simulink model "ROBOT_OK"  (R2021a)
settings: Solver=FixedStepAuto  StartTime=0.0  StopTime=inf  FixedStep=0.001  RelTol=1e-3
model workspace: external: MATLAB File E:\2024\TINH_TOAN_ROBOT_6_DOF\ROBOT_OK_DataFile.m (data not in the file)
values from neighbouring files (symbols this model uses):
  X = Toado(:,1)    [QuydaoK.m]
  Y = Toado(:,2)    [QuydaoK.m]
  Z = Toado(:,3)    [QuydaoK.m]
undefined symbols (not defined in the file or in its folder): smiData
libraries: sm_lib x38, nesl_utility x30, sharedutil x16, sharedtransform x12, dspmtrx3 x12, simulink_extras x8, pid_lib x6, simulink x3
(part 2 of 6)

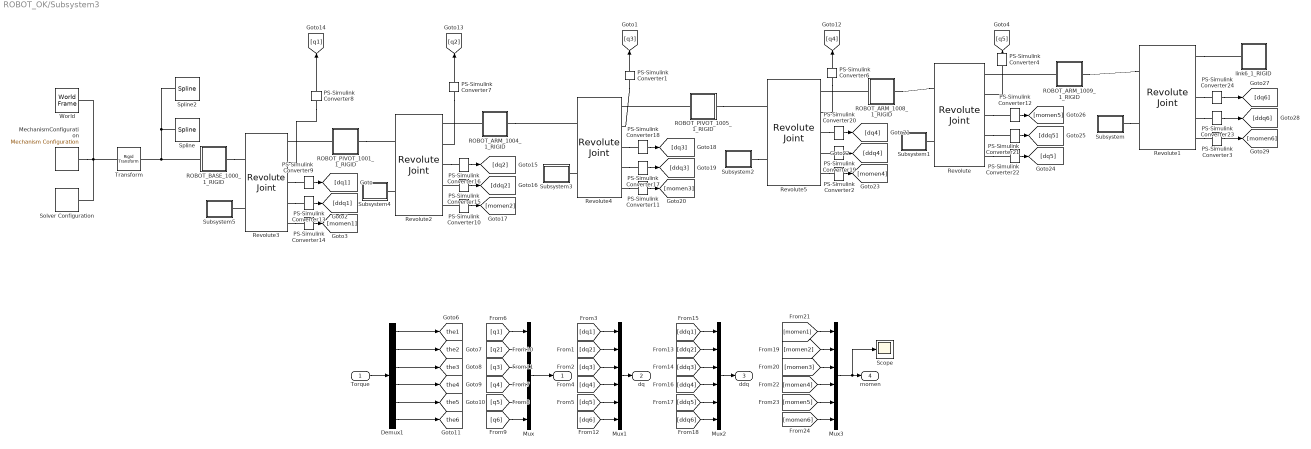
== system ROBOT_OK/Subsystem3 ==
  Torque : Inport
  Demux1 : Demux  Outputs=6
  MechanismConfiguration : sm_lib/Utilities/Mechanism Configuration  UniformGravity=Constant  GravityVector=[0 -9.80665 0]  GravityVectorUnits=m/s^2  GravityUnits=m/s^2  LinearizationDelta=0.001  JointModeTransitionNonlinearIterations=2
  Mux{,1..3} (4 alike) : Mux  Inputs=6
  PS-Simulink Converter{1..4,6..24} (23 alike) : nesl_utility/PS-Simulink Converter  PhysicalDomain=network_engine_domain  SubClassName=ps_output  LeftPortType=input  RightPortType=output  PseudoPeriodic=off  Frequencies=[]  Unit=inherit  AffineConversion=off
      settings: SourceProductBaseCode=PW,SS
  ROBOT_ARM_1004_1_RIGID : Subsystem
  ROBOT_ARM_1008_1_RIGID : Subsystem
  ROBOT_ARM_1009_1_RIGID : Subsystem
  ROBOT_BASE_1000_1_RIGID : Subsystem
  ROBOT_PIVOT_1001_1_RIGID : Subsystem
  ROBOT_PIVOT_1005_1_RIGID : Subsystem
  Revolute : sm_lib/Joints/Revolute Joint  JointMode=Normal  SenseConstraintForce=off  SenseConstraintForceX=off  SenseConstraintForceY=off  SenseConstraintForceZ=off  SenseConstraintTorque=off  SenseConstraintTorqueX=off  SenseConstraintTorqueY=off  SenseConstraintTorqueZ=off  SenseTotalForce=off  SenseTotalForceX=off  SenseTotalForceY=off  SenseTotalForceZ=off  SenseTotalTorque=off  SenseTotalTorqueX=off  SenseTotalTorqueY=off  SenseTotalTorqueZ=off  CompositeWrenchDir=FollowerOnBase  CompositeWrenchFrame=BaseFrame  EquilibriumPosition=0  EquilibriumPositionUnits=deg  SpringStiffness=0  SpringStiffnessUnits=N*m/deg  DampingCoefficient=0  DampingCoefficientUnits=N*m/(deg/s)  TorqueActuationMode=ComputedTorque  MotionActuationMode=InputMotion  SensePosition=on  SenseVelocity=on  SenseAcceleration=on  SenseTorqueForce=on  SenseLowerLimitTorqueForce=off  SenseUpperLimitTorqueForce=off  LowerLimitSpecify=off  LowerLimitBound=-90  LowerLimitBoundUnits=deg  LowerLimitStiffness=1e4  LowerLimitStiffnessUnits=N*m/deg  LowerLimitDamping=10  LowerLimitDampingUnits=N*m/(deg/s)  LowerLimitTransitionRegionWidth=0.1  LowerLimitTransitionRegionWidthUnits=deg  UpperLimitSpecify=off  UpperLimitBound=90  UpperLimitBoundUnits=deg  UpperLimitStiffness=1e4  UpperLimitStiffnessUnits=N*m/deg  UpperLimitDamping=10  UpperLimitDampingUnits=N*m/(deg/s)  UpperLimitTransitionRegionWidth=0.1  UpperLimitTransitionRegionWidthUnits=deg  PositionTargetSpecify=on  PositionTargetPriority=Low  PositionTargetValue=smiData.RevoluteJoint(1).Rz.Pos  PositionTargetValueUnits=deg  VelocityTargetSpecify=off  VelocityTargetPriority=High  VelocityTargetValue=0  VelocityTargetValueUnits=deg/s
  Revolute1 : sm_lib/Joints/Revolute Joint  JointMode=Normal  SenseConstraintForce=off  SenseConstraintForceX=off  SenseConstraintForceY=off  SenseConstraintForceZ=off  SenseConstraintTorque=off  SenseConstraintTorqueX=off  SenseConstraintTorqueY=off  SenseConstraintTorqueZ=off  SenseTotalForce=off  SenseTotalForceX=off  SenseTotalForceY=off  SenseTotalForceZ=off  SenseTotalTorque=off  SenseTotalTorqueX=off  SenseTotalTorqueY=off  SenseTotalTorqueZ=off  CompositeWrenchDir=FollowerOnBase  CompositeWrenchFrame=BaseFrame  EquilibriumPosition=0  EquilibriumPositionUnits=deg  SpringStiffness=0  SpringStiffnessUnits=N*m/deg  DampingCoefficient=0  DampingCoefficientUnits=N*m/(deg/s)  TorqueActuationMode=ComputedTorque  MotionActuationMode=InputMotion  SensePosition=on  SenseVelocity=on  SenseAcceleration=on  SenseTorqueForce=on  SenseLowerLimitTorqueForce=off  SenseUpperLimitTorqueForce=off  LowerLimitSpecify=off  LowerLimitBound=-90  LowerLimitBoundUnits=deg  LowerLimitStiffness=1e4  LowerLimitStiffnessUnits=N*m/deg  LowerLimitDamping=10  LowerLimitDampingUnits=N*m/(deg/s)  LowerLimitTransitionRegionWidth=0.1  LowerLimitTransitionRegionWidthUnits=deg  UpperLimitSpecify=off  UpperLimitBound=90  UpperLimitBoundUnits=deg  UpperLimitStiffness=1e4  UpperLimitStiffnessUnits=N*m/deg  UpperLimitDamping=10  UpperLimitDampingUnits=N*m/(deg/s)  UpperLimitTransitionRegionWidth=0.1  UpperLimitTransitionRegionWidthUnits=deg  PositionTargetSpecify=on  PositionTargetPriority=Low  PositionTargetValue=smiData.RevoluteJoint(2).Rz.Pos  PositionTargetValueUnits=deg  VelocityTargetSpecify=off  VelocityTargetPriority=High  VelocityTargetValue=0  VelocityTargetValueUnits=deg/s
  Revolute2 : sm_lib/Joints/Revolute Joint  JointMode=Normal  SenseConstraintForce=off  SenseConstraintForceX=off  SenseConstraintForceY=off  SenseConstraintForceZ=off  SenseConstraintTorque=off  SenseConstraintTorqueX=off  SenseConstraintTorqueY=off  SenseConstraintTorqueZ=off  SenseTotalForce=off  SenseTotalForceX=off  SenseTotalForceY=off  SenseTotalForceZ=off  SenseTotalTorque=off  SenseTotalTorqueX=off  SenseTotalTorqueY=off  SenseTotalTorqueZ=off  CompositeWrenchDir=FollowerOnBase  CompositeWrenchFrame=BaseFrame  EquilibriumPosition=0  EquilibriumPositionUnits=deg  SpringStiffness=0  SpringStiffnessUnits=N*m/deg  DampingCoefficient=0  DampingCoefficientUnits=N*m/(deg/s)  TorqueActuationMode=ComputedTorque  MotionActuationMode=InputMotion  SensePosition=on  SenseVelocity=on  SenseAcceleration=on  SenseTorqueForce=on  SenseLowerLimitTorqueForce=off  SenseUpperLimitTorqueForce=off  LowerLimitSpecify=off  LowerLimitBound=-90  LowerLimitBoundUnits=deg  LowerLimitStiffness=1e4  LowerLimitStiffnessUnits=N*m/deg  LowerLimitDamping=10  LowerLimitDampingUnits=N*m/(deg/s)  LowerLimitTransitionRegionWidth=0.1  LowerLimitTransitionRegionWidthUnits=deg  UpperLimitSpecify=off  UpperLimitBound=90  UpperLimitBoundUnits=deg  UpperLimitStiffness=1e4  UpperLimitStiffnessUnits=N*m/deg  UpperLimitDamping=10  UpperLimitDampingUnits=N*m/(deg/s)  UpperLimitTransitionRegionWidth=0.1  UpperLimitTransitionRegionWidthUnits=deg  PositionTargetSpecify=on  PositionTargetPriority=Low  PositionTargetValue=smiData.RevoluteJoint(3).Rz.Pos  PositionTargetValueUnits=deg  VelocityTargetSpecify=off  VelocityTargetPriority=High  VelocityTargetValue=0  VelocityTargetValueUnits=deg/s
  Revolute3 : sm_lib/Joints/Revolute Joint  JointMode=Normal  SenseConstraintForce=off  SenseConstraintForceX=off  SenseConstraintForceY=off  SenseConstraintForceZ=off  SenseConstraintTorque=off  SenseConstraintTorqueX=off  SenseConstraintTorqueY=off  SenseConstraintTorqueZ=off  SenseTotalForce=off  SenseTotalForceX=off  SenseTotalForceY=off  SenseTotalForceZ=off  SenseTotalTorque=off  SenseTotalTorqueX=off  SenseTotalTorqueY=off  SenseTotalTorqueZ=off  CompositeWrenchDir=FollowerOnBase  CompositeWrenchFrame=BaseFrame  EquilibriumPosition=0  EquilibriumPositionUnits=deg  SpringStiffness=0  SpringStiffnessUnits=N*m/deg  DampingCoefficient=0  DampingCoefficientUnits=N*m/(deg/s)  TorqueActuationMode=ComputedTorque  MotionActuationMode=InputMotion  SensePosition=on  SenseVelocity=on  SenseAcceleration=on  SenseTorqueForce=on  SenseLowerLimitTorqueForce=off  SenseUpperLimitTorqueForce=off  LowerLimitSpecify=off  LowerLimitBound=-90  LowerLimitBoundUnits=deg  LowerLimitStiffness=1e4  LowerLimitStiffnessUnits=N*m/deg  LowerLimitDamping=10  LowerLimitDampingUnits=N*m/(deg/s)  LowerLimitTransitionRegionWidth=0.1  LowerLimitTransitionRegionWidthUnits=deg  UpperLimitSpecify=off  UpperLimitBound=90  UpperLimitBoundUnits=deg  UpperLimitStiffness=1e4  UpperLimitStiffnessUnits=N*m/deg  UpperLimitDamping=10  UpperLimitDampingUnits=N*m/(deg/s)  UpperLimitTransitionRegionWidth=0.1  UpperLimitTransitionRegionWidthUnits=deg  PositionTargetSpecify=on  PositionTargetPriority=Low  PositionTargetValue=smiData.RevoluteJoint(4).Rz.Pos  PositionTargetValueUnits=deg  VelocityTargetSpecify=off  VelocityTargetPriority=High  VelocityTargetValue=0  VelocityTargetValueUnits=deg/s
  Revolute4 : sm_lib/Joints/Revolute Joint  JointMode=Normal  SenseConstraintForce=off  SenseConstraintForceX=off  SenseConstraintForceY=off  SenseConstraintForceZ=off  SenseConstraintTorque=off  SenseConstraintTorqueX=off  SenseConstraintTorqueY=off  SenseConstraintTorqueZ=off  SenseTotalForce=off  SenseTotalForceX=off  SenseTotalForceY=off  SenseTotalForceZ=off  SenseTotalTorque=off  SenseTotalTorqueX=off  SenseTotalTorqueY=off  SenseTotalTorqueZ=off  CompositeWrenchDir=FollowerOnBase  CompositeWrenchFrame=BaseFrame  EquilibriumPosition=0  EquilibriumPositionUnits=deg  SpringStiffness=0  SpringStiffnessUnits=N*m/deg  DampingCoefficient=0  DampingCoefficientUnits=N*m/(deg/s)  TorqueActuationMode=ComputedTorque  MotionActuationMode=InputMotion  SensePosition=on  SenseVelocity=on  SenseAcceleration=on  SenseTorqueForce=on  SenseLowerLimitTorqueForce=off  SenseUpperLimitTorqueForce=off  LowerLimitSpecify=off  LowerLimitBound=-90  LowerLimitBoundUnits=deg  LowerLimitStiffness=1e4  LowerLimitStiffnessUnits=N*m/deg  LowerLimitDamping=10  LowerLimitDampingUnits=N*m/(deg/s)  LowerLimitTransitionRegionWidth=0.1  LowerLimitTransitionRegionWidthUnits=deg  UpperLimitSpecify=off  UpperLimitBound=90  UpperLimitBoundUnits=deg  UpperLimitStiffness=1e4  UpperLimitStiffnessUnits=N*m/deg  UpperLimitDamping=10  UpperLimitDampingUnits=N*m/(deg/s)  UpperLimitTransitionRegionWidth=0.1  UpperLimitTransitionRegionWidthUnits=deg  PositionTargetSpecify=on  PositionTargetPriority=Low  PositionTargetValue=smiData.RevoluteJoint(5).Rz.Pos  PositionTargetValueUnits=deg  VelocityTargetSpecify=off  VelocityTargetPriority=High  VelocityTargetValue=0  VelocityTargetValueUnits=deg/s
  Revolute5 : sm_lib/Joints/Revolute Joint  JointMode=Normal  SenseConstraintForce=off  SenseConstraintForceX=off  SenseConstraintForceY=off  SenseConstraintForceZ=off  SenseConstraintTorque=off  SenseConstraintTorqueX=off  SenseConstraintTorqueY=off  SenseConstraintTorqueZ=off  SenseTotalForce=off  SenseTotalForceX=off  SenseTotalForceY=off  SenseTotalForceZ=off  SenseTotalTorque=off  SenseTotalTorqueX=off  SenseTotalTorqueY=off  SenseTotalTorqueZ=off  CompositeWrenchDir=FollowerOnBase  CompositeWrenchFrame=BaseFrame  EquilibriumPosition=0  EquilibriumPositionUnits=deg  SpringStiffness=0  SpringStiffnessUnits=N*m/deg  DampingCoefficient=0  DampingCoefficientUnits=N*m/(deg/s)  TorqueActuationMode=ComputedTorque  MotionActuationMode=InputMotion  SensePosition=on  SenseVelocity=on  SenseAcceleration=on  SenseTorqueForce=on  SenseLowerLimitTorqueForce=off  SenseUpperLimitTorqueForce=off  LowerLimitSpecify=off  LowerLimitBound=-90  LowerLimitBoundUnits=deg  LowerLimitStiffness=1e4  LowerLimitStiffnessUnits=N*m/deg  LowerLimitDamping=10  LowerLimitDampingUnits=N*m/(deg/s)  LowerLimitTransitionRegionWidth=0.1  LowerLimitTransitionRegionWidthUnits=deg  UpperLimitSpecify=off  UpperLimitBound=90  UpperLimitBoundUnits=deg  UpperLimitStiffness=1e4  UpperLimitStiffnessUnits=N*m/deg  UpperLimitDamping=10  UpperLimitDampingUnits=N*m/(deg/s)  UpperLimitTransitionRegionWidth=0.1  UpperLimitTransitionRegionWidthUnits=deg  PositionTargetSpecify=on  PositionTargetPriority=Low  PositionTargetValue=smiData.RevoluteJoint(6).Rz.Pos  PositionTargetValueUnits=deg  VelocityTargetSpecify=off  VelocityTargetPriority=High  VelocityTargetValue=0  VelocityTargetValueUnits=deg/s
  Scope : Scope
  Solver Configuration : nesl_utility/Solver Configuration  PhysicalDomain=network_engine_domain  SubClassName=solver  LeftPortType=input  RightPortType=generic  Tones=[]  Harmonics=[]  SimulateNoise=off  Profile=off  UseLocalSampling=off  EnableSwitchedLinearOptims=on  FrequencyDomain=off  UseCCode=off  RelTol=0.001  AbsTol=1e-06  MinStep=1e-09  ToWorkspace=off  RevertToSquareIcSolve=off  NumHomotopyIterations=100  PhasorMode=off  PhasorModeNumHarmonics=1  DoDC=off  ResidualTolerance=1e-09  UseLocalSolver=off  LocalSolverChoice=NE_BACKWARD_EULER_ADVANCER  LocalSolverSampleTime=0.001  DoFixedCost=off  MaxNonlinIter=3  MaxModeIter=2  ComputeImpulses=off  ImpulseIterations=2  LinearAlgebra=auto  EquationFormulation=NE_TIME_EF  DelaysMemoryBudget=1024  AutomaticFiltering=on  FilteringTimeConstant=0.001  PartitionStorageMethod=AS_NEEDED  PartitionMemoryBudget=1024  PartitionMethod=ROBUST
      settings: SourceProductBaseCode=PW,SS
  Spline : sm_lib/Curves and Surfaces/Spline  GraphicAmbientColor=[0.15 0.15 0.15 1.0]  GraphicDiffuseColor=[1.0 0.2 0.2]  DataPoints=|  DataPointsUnits=mm  GraphicEmissiveColor=[0.0 0.0 0.0 1.0]  EndConditionType=Natural  MarkerShape=Sphere  MarkerSize=10  GraphicType=FromGeometry  GraphicOpacity=1.0  GraphicShininess=75  GraphicSpecularColor=[0.5 0.5 0.5 1.0]  GraphicVisPropType=SimpleVisualProperties
      | [0	1246.42	935;
      | 0	1141.996516	911.946802530624;
      | 0	1041.84119	877.504979796037;
      | 0	947.4760988	832.945432411482;
      | 0	860.2282809	780.049364286457;
      | 0	781.0917361	721.088113877702;
      | 0	710.6207008	658.738466752562;
      | 0	648.8850879	595.949836689254;
      | 0	595.5043466	535.787921681756;
      | 0	549.759162	481.278705653943;
      | 0	510.7655072	435.268882540223;
      | 0	477.6849723	400.307708228352;
      | 0	449.9395711	378.545189126439;
      | 0	427.397846	371.635894428904;
      | 0	410.5013013	380.638467275163;
      | 0	400.3057691	405.90807653484;
      | 0	398.4216033	446.990560698198;
      | 0	406.8500062	502.53916250366;
      | 0	427.7297913	570.282947538006;
      | 0	463.0271933	647.07604555658;
      | 0	514.2167348	729.046527199941;
      | 0	582.0084683	811.844148723031;
      | 0	666.1719718	890.962242341668;
      | 0	765.4893384	962.088242116838;
      | 0	877.8417585	1021.42733844735;
      | 0	1000.404901	1065.9490660948;
      | 0	1129.90644	1093.52633771776;
      | 0	1262.891818	1102.96405231642;
      | 0	1395.95343	1093.94028862832;
      | 0	1525.899432	1066.8984206983;
      | 0	1649.862571	1022.92897322416;
      | 0	1765.367549	963.6674944662;
      | 0	1870.381646	891.215898833618;
      | 0	1963.36719	808.077974683463;
      | 0	2043.340473	717.091385577582;
      | 0	2109.926876	621.340482052643;
      | 0	2163.392348	524.044061250851;
      | 0	2204.630239	428.4245921448;
      | 0	2235.089177	337.574886372955;
      | 0	2256.639117	254.341183574269;
      | 0	2271.38475	181.237472054488;
      | 0	2281.444993	120.396534357569;
      | 0	2288.72268	73.5521764178257;
      | 0	2294.690175	42.0380828695401;
      | 0	2300.215416	26.7846353299187;
      | 0	2305.450033	28.2972912781336;
      | 0	2309.796901	46.6085230636865;
      | 0	2311.968166	81.2079655344927;
      | 0	2310.135307	130.968983543269;
      | 0	2302.159813	194.100113783151;
      | 0	2285.877616	268.152603742306;
      | 0	2259.396091	350.107874126506;
      | 0	2221.353866	436.551381778171;
      | 0	2171.095961	523.915981686465;
      | 0	2108.73191	608.755590151463;
      | 0	2035.070597	687.996902364093;
      | 0	1951.455626	759.119138486728;
      | 0	1859.549516	820.230221821996;
      | 0	1761.125197	870.037149990835;
      | 0	1657.915028	907.738656326344;
      | 0	1551.543597	932.888783065801;
      | 0	1443.539645	945.283506254234;
      | 0	1335.395716	944.908427869492;
      | 0	1228.630725	931.95979110792;
      | 0	1124.81432	906.923588170289;
      | 0	1025.529695	870.677954638411;
      | 0	932.2759657	824.578104589049;
      | 0	846.3334325	770.490930605497;
      | 0	768.6282406	710.76345131364;
      | 0	699.6342812	648.128548458328;
      | 0	639.3411388	585.566383309259;
      | 0	587.3015276	526.146582842937;
      | 0	542.7549079	472.874162497067;
      | 0	504.8096775	428.553512354063;
      | 0	472.6565643	395.673576138863;
      | 0	445.780909	376.30779818038;
      | 0	424.1407935	372.017784899407;
      | 0	408.2807426	383.751546181202;
      | 0	399.3568911	411.735273009936;
      | 0	399.0594768	455.369520441295;]
  Spline2 : sm_lib/Curves and Surfaces/Spline  GraphicAmbientColor=[0.15 0.15 0.15 1.0]  GraphicDiffuseColor=[0 0 0]  DataPoints=|  DataPointsUnits=mm  GraphicEmissiveColor=[0.0 0.0 0.0 1.0]  EndConditionType=Natural  MarkerShape=Sphere  MarkerSize=10  GraphicType=FromGeometry  GraphicOpacity=1.0  GraphicShininess=75  GraphicSpecularColor=[0.5 0.5 0.5 1.0]  GraphicVisPropType=SimpleVisualProperties
      | [935	1810.42	0;
      | 889.3889292	1810.42	288.465479096214;
      | 758.7217457	1810.42	546.412218637785;
      | 560.1702039	1810.42	748.621628529161;
      | 318.3269723	1810.42	879.143298173723;
      | 60.39312617	1810.42	933.047517713805;
      | -188.5776271	1810.42	915.785716505588;
      | -409.2782548	1810.42	840.664207718416;
      | -589.9869882	1810.42	725.355329330757;
      | -726.6195992	1810.42	588.429229419664;
      | -821.4195772	1810.42	446.648495104488;
      | -880.9185172	1810.42	313.380864314407;
      | -913.7700293	1810.42	198.114445450209;
      | -928.8792176	1810.42	106.810108028732;
      | -934.02333	1810.42	42.7249224223983;
      | -934.9710466	1810.42	7.35812317060034;
      | -934.9991611	1810.42	1.25249341683292;
      | -934.6794561	1810.42	24.4808972224464;
      | -931.8460187	1810.42	76.7332882394875;
      | -921.7261092	1810.42	156.990380392949;
      | -897.2966469	1810.42	262.837834788631;
      | -849.9841137	1810.42	389.553599012022;
      | -770.8291947	1810.42	529.195004386879;
      | -652.1644528	1810.42	670.004870485479;
      | -489.6956927	1810.42	796.506828922027;
      | -284.6593243	1810.42	890.6144334594;
      | -45.5155654	1810.42	933.891499750544;
      | 211.4678954	1810.42	910.772380583934;
      | 463.2840896	1810.42	812.15321970817;
      | 683.0932046	1810.42	638.442380960117;
      | 844.6072888	1810.42	401.077957159677;
      | 927.0338861	1810.42	121.791518640453;
      | 919.3214855	1810.42	-170.508082741636;
      | 822.5162353	1810.42	-444.625733276075;
      | 649.5361157	1810.42	-672.553220458847;
      | 422.4299451	1810.42	-834.133047850261;
      | 167.9237268	1810.42	-919.797054783009;
      | -87.51207951	1810.42	-930.895609582728;
      | -321.8492458	1810.42	-877.859933587599;
      | -520.10804	1810.42	-776.989463694896;
      | -675.1219042	1810.42	-646.865839625697;
      | -786.7233499	1810.42	-505.26366447985;
      | -859.9283141	1810.42	-367.080773854093;
      | -902.7588492	1810.42	-243.416228168219;
      | -924.2130658	1810.42	-141.616415037239;
      | -932.6713587	1810.42	-65.9479851689328;
      | -934.8163514	1810.42	-18.5307640159085;
      | -934.9999728	1810.42	-0.225422394920873;
      | -934.9321273	1810.42	-11.2657637128891;
      | -933.579647	1810.42	-51.5174025001901;
      | -927.2259183	1810.42	-120.320805981722;
      | -909.7215411	1810.42	-215.943783693215;
      | -873.0253473	1810.42	-334.741307447926;
      | -808.1637472	1810.42	-470.208844819455;
      | -706.6974329	1810.42	-612.21216771785;
      | -562.6613179	1810.42	-746.751124072799;
      | -374.7449343	1810.42	-856.616153375299;
      | -148.2547974	1810.42	-923.171444020766;
      | 103.7629974	1810.42	-929.224537116843;
      | 360.8552747	1810.42	-862.559256347886;
      | 597.3133262	1810.42	-719.334268874758;
      | 786.0247841	1810.42	-506.349719830471;]
  Subsystem : Subsystem
  Subsystem1 : Subsystem
  Subsystem2 : Subsystem
  Subsystem3 : Subsystem
  Subsystem4 : Subsystem
  Subsystem5 : Subsystem
  Transform : sm_lib/Frames and Transforms/Rigid Transform  TranslationMethod=Cartesian  TranslationStandardOffset=0  TranslationLengthUnit=mm  TranslationStandardAxis=+Z  TranslationCartesianOffset=smiData.RigidTransform(6).translation  TranslationROffset=0  TranslationROffsetUnits=m  TranslationZOffset=0  TranslationZOffsetUnits=m  TranslationThetaOffset=0  TranslationThetaOffsetUnits=deg  RotationMethod=ArbitraryAxis  RotationAngleUnits=rad  RotationStandardAxis=+Z  RotationAngle=smiData.RigidTransform(6).angle  RotationArbitraryAxis=smiData.RigidTransform(6).axis  FollAlignAxisA=+X  BaseAlignAxisA=+Y  FollAlignAxisB=+Y  BaseAlignAxisB=+Z  RotationSequenceAxes=FollowerAxes  RotationSequence=XYX  RotationSequenceAngles=[0 0 0]  RotationSequenceAnglesUnits=deg  RotationMatrix=[1 0 0; 0 1 0; 0 0 1]
  World : sm_lib/Frames and Transforms/World Frame
  link6_1_RIGID : Subsystem
  q : Outport
  dq : Outport  Port=2
  ddq : Outport  Port=3
  momen : Outport  Port=4
  tag scope: the1=global, the2=global, the3=global, the4=global, the5=global, the6=global
  wires:
  [ddq3] -> Mux2/3
  [ddq1] -> Mux2/1
  [q1] -> Mux/1
  [ddq6] -> Mux2/6
  Mux2/1 -> ddq/1
  PS-Simulink Converter22/1 -> [dq5]
  PS-Simulink Converter13/1 -> [ddq1]
  [momen1] -> Mux3/1
  [dq4] -> Mux1/4
  [ddq2] -> Mux2/2
  PS-Simulink Converter3/1 -> [momen6]
  Mux/1 -> q/1
  [ddq4] -> Mux2/4
  PS-Simulink Converter21/1 -> [ddq5]
  Mux3/1 -> Scope/1, momen/1
  [ddq5] -> Mux2/5
  Demux1/3 -> [the3]
  PS-Simulink Converter19/1 -> [ddq4]
  PS-Simulink Converter18/1 -> [dq3]
  PS-Simulink Converter20/1 -> [dq4]
  PS-Simulink Converter17/1 -> [ddq3]
  PS-Simulink Converter24/1 -> [dq6]
  PS-Simulink Converter23/1 -> [ddq6]
  PS-Simulink Converter14/1 -> [momen1]
  PS-Simulink Converter2/1 -> [momen4]
  Demux1/6 -> [the6]
  PS-Simulink Converter12/1 -> [momen5]
  [dq3] -> Mux1/3
  [momen6] -> Mux3/6
  [momen3] -> Mux3/3
  [dq5] -> Mux1/5
  [dq1] -> Mux1/1
  [momen5] -> Mux3/5
  [momen2] -> Mux3/2
  Demux1/4 -> [the4]
  PS-Simulink Converter4/1 -> [q5]
  Mux1/1 -> dq/1
  PS-Simulink Converter7/1 -> [q2]
  [dq2] -> Mux1/2
  PS-Simulink Converter8/1 -> [q1]
  PS-Simulink Converter15/1 -> [ddq2]
  Demux1/2 -> [the2]
  [dq6] -> Mux1/6
  PS-Simulink Converter11/1 -> [momen3]
  PS-Simulink Converter6/1 -> [q4]
  PS-Simulink Converter1/1 -> [q3]
  [q5] -> Mux/5
  PS-Simulink Converter16/1 -> [dq2]
  [q4] -> Mux/4
  Demux1/5 -> [the5]
  [q2] -> Mux/2
  Demux1/1 -> [the1]
  Torque/1 -> Demux1/1
  PS-Simulink Converter10/1 -> [momen2]
  [q6] -> Mux/6
  PS-Simulink Converter9/1 -> [dq1]
  [q3] -> Mux/3
  [momen4] -> Mux3/4
  connections:
  Revolute3/RConn4 -- PS-Simulink Converter13/LConn1
  Subsystem/RConn1 -- Revolute1/LConn2
  Revolute1/RConn3 -- PS-Simulink Converter24/LConn1
  Revolute5/RConn4 -- PS-Simulink Converter19/LConn1
  Subsystem4/RConn1 -- Revolute2/LConn2
  Revolute4/RConn4 -- PS-Simulink Converter17/LConn1
  PS-Simulink Converter10/LConn1 -- Revolute2/RConn5
  Subsystem1/RConn1 -- Revolute/LConn2
  Revolute5/RConn3 -- PS-Simulink Converter20/LConn1
  Revolute1/RConn5 -- PS-Simulink Converter3/LConn1
  Revolute3/RConn5 -- PS-Simulink Converter14/LConn1
  Revolute1/RConn4 -- PS-Simulink Converter23/LConn1
  PS-Simulink Converter8/LConn1 -- Revolute3/RConn2
  Revolute3/RConn3 -- PS-Simulink Converter9/LConn1
  Revolute4/RConn5 -- PS-Simulink Converter11/LConn1
  Revolute4/RConn3 -- PS-Simulink Converter18/LConn1
  PS-Simulink Converter7/LConn1 -- Revolute2/RConn2
  PS-Simulink Converter6/LConn1 -- Revolute5/RConn2
  PS-Simulink Converter15/LConn1 -- Revolute2/RConn4
  Revolute3/LConn2 -- Subsystem5/RConn1
  Revolute2/RConn3 -- PS-Simulink Converter16/LConn1
  Revolute5/RConn5 -- PS-Simulink Converter2/LConn1
  PS-Simulink Converter4/LConn1 -- Revolute/RConn2
  Revolute4/LConn2 -- Subsystem3/RConn1
  PS-Simulink Converter1/LConn1 -- Revolute4/RConn2
  Solver Configuration/RConn1 -- Transform/LConn1 -- World/RConn1 -- MechanismConfiguration/RConn1
  ROBOT_PIVOT_1001_1_RIGID/RConn1 -- Revolute2/LConn1
  ROBOT_PIVOT_1005_1_RIGID/LConn1 -- Revolute4/RConn1
  ROBOT_ARM_1008_1_RIGID/RConn1 -- Revolute/LConn1
  ROBOT_ARM_1008_1_RIGID/LConn1 -- Revolute5/RConn1
  ROBOT_ARM_1004_1_RIGID/LConn1 -- Revolute2/RConn1
  Revolute1/RConn1 -- link6_1_RIGID/LConn1
  ROBOT_PIVOT_1001_1_RIGID/LConn1 -- Revolute3/RConn1
  ROBOT_ARM_1004_1_RIGID/RConn1 -- Revolute4/LConn1
  ROBOT_BASE_1000_1_RIGID/RConn1 -- Revolute3/LConn1
  ROBOT_ARM_1009_1_RIGID/LConn1 -- Revolute/RConn1
  ROBOT_BASE_1000_1_RIGID/LConn1 -- Transform/RConn1 -- Spline/LConn1 -- Spline2/LConn1
  ROBOT_ARM_1009_1_RIGID/RConn1 -- Revolute1/LConn1
  ROBOT_PIVOT_1005_1_RIGID/RConn1 -- Revolute5/LConn1
  Subsystem2/RConn1 -- Revolute5/LConn2
  Revolute/RConn5 -- PS-Simulink Converter22/LConn1
  Revolute/RConn4 -- PS-Simulink Converter21/LConn1
  Revolute/RConn3 -- PS-Simulink Converter12/LConn1

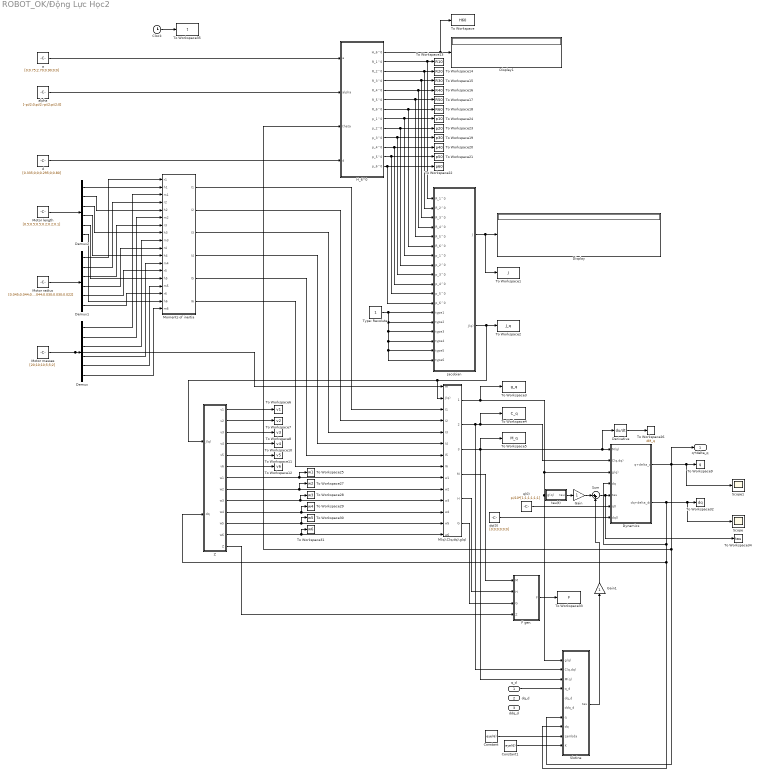
== system ROBOT_OK/Động Lực Học2 ==
  q_d : Inport
  dq_d : Inport  Port=2
  ddq_d : Inport  Port=3
  Clock : Clock
  Constant : Constant  Value=eye(6)
  Constant1 : Constant  Value=eye(6)
  Demux : Demux  Outputs=6
  Demux1 : Demux  Outputs=6
  Demux2 : Demux  Outputs=6
  Derivative : Derivative
  Display : Display
  Display1 : Display
  Dynamics : Subsystem
  F gen. : Subsystem
  Gain : Gain
  Gain1 : Gain
  H_6^0 : Subsystem
  Jacobian : Subsystem
  M(q),C(q,dq),g(q) : Subsystem
  Moments of inertia : Subsystem
  Motor length : Constant  Value=[0.5;0.5;0.5;0.2;0.2;0.1]
  Motor masses : Constant  Value=[20;10;10;5;5;2]
  Motor radius : Constant  Value=[0.045;0.044;0.044;0.030;0.030;0.022]  VectorParams1D=off
  Scope : Scope
  Scope1 : Scope
  Slotine : Subsystem
  Sum : Sum  Inputs=|++
  To Workspace : ToWorkspace  VariableName=H60  SampleTime=-1
  To Workspace1 : ToWorkspace  VariableName=J  SampleTime=-1
  To Workspace10 : ToWorkspace  VariableName=v4  SampleTime=-1
  To Workspace11 : ToWorkspace  VariableName=v5  SampleTime=-1
  To Workspace12 : ToWorkspace  VariableName=v6  SampleTime=-1
  To Workspace13 : ToWorkspace  VariableName=R10  SampleTime=-1
  To Workspace14 : ToWorkspace  VariableName=R20  SampleTime=-1
  To Workspace15 : ToWorkspace  VariableName=R30  SampleTime=-1
  To Workspace16 : ToWorkspace  VariableName=R40  SampleTime=-1
  To Workspace17 : ToWorkspace  VariableName=R50  SampleTime=-1
  To Workspace18 : ToWorkspace  VariableName=R60  SampleTime=-1
  To Workspace19 : ToWorkspace  VariableName=p30  SampleTime=-1
  To Workspace2 : ToWorkspace  VariableName=J_q  SampleTime=-1
  To Workspace20 : ToWorkspace  VariableName=p40  SampleTime=-1
  To Workspace21 : ToWorkspace  VariableName=p50  SampleTime=-1
  To Workspace22 : ToWorkspace  VariableName=p60  SampleTime=-1
  To Workspace23 : ToWorkspace  VariableName=p20  SampleTime=-1
  To Workspace24 : ToWorkspace  VariableName=p10  SampleTime=-1
  To Workspace25 : ToWorkspace  VariableName=w1  SampleTime=-1
  To Workspace26 : ToWorkspace  VariableName=dM_q  SampleTime=-1
  To Workspace27 : ToWorkspace  VariableName=w2  SampleTime=-1
  To Workspace28 : ToWorkspace  VariableName=w3  SampleTime=-1
  To Workspace29 : ToWorkspace  VariableName=w4  SampleTime=-1
  To Workspace3 : ToWorkspace  VariableName=g_q  SampleTime=-1
  To Workspace30 : ToWorkspace  VariableName=w5  SampleTime=-1
  To Workspace31 : ToWorkspace  VariableName=w6  SampleTime=-1
  To Workspace32 : ToWorkspace  VariableName=dq  SampleTime=-1
  To Workspace33 : ToWorkspace  VariableName=F  SampleTime=-1
  To Workspace34 : ToWorkspace  VariableName=tau  SampleTime=-1
  To Workspace35 : ToWorkspace  VariableName=t  SampleTime=-1
  To Workspace4 : ToWorkspace  VariableName=C_q  SampleTime=-1
  To Workspace5 : ToWorkspace  VariableName=M_q  SampleTime=-1
  To Workspace6 : ToWorkspace  VariableName=v1  SampleTime=-1
  To Workspace7 : ToWorkspace  VariableName=v2  SampleTime=-1
  To Workspace8 : ToWorkspace  VariableName=v3  SampleTime=-1
  To Workspace9 : ToWorkspace  VariableName=q  SampleTime=-1
  Type: Revolute : Constant
  Z : Subsystem
  a : Constant  Value=[0;0.75;2.70;0.90;0;0]
  alpha : Constant  Value=[-pi/2;0;pi/2;-pi/2;pi/2;0]
  d : Constant  Value=[0.335;0;0;0.295;0;0.80]
  dq(0) : Constant  Value=[0;0;0;0;0;0]
  q(0) : Constant  Value=pi/10*[1;1;1;1;1;1]
  tau(t) : Subsystem
  q+delta_q : Outport
  wires:
  Slotine/1(tau) -> Gain1/1
  Z/13(Z) -> F gen./4(Z)
  M(q),C(q,dq),g(q)/1(g(q)) -> Dynamics/3(g(q)), tau(t)/1(g(q)), Slotine/1(g(q)), To Workspace3/1
  Demux/4 -> Moments of inertia/12(m4)
  Motor radius/1 -> Demux1/1
  Gain1/1 -> Sum/2
  Demux/5 -> Moments of inertia/15(m5)
  Moments of inertia/5(I5) -> M(q),C(q,dq),g(q)/7(I5)
  Motor length/1 -> Demux2/1
  Z/3(v3) -> To Workspace8/1
  Gain/1 -> Sum/1
  H_6^0/3(R_2^0) -> To Workspace14/1, Jacobian/2(R_2^0)
  Jacobian/1(J) -> To Workspace1/1, Display/1
  Constant/1 -> Slotine/9(Lambda)
  Motor masses/1 -> Demux/1, M(q),C(q,dq),g(q)/1(m)
  Demux2/6 -> Moments of inertia/17(h6)
  Demux1/6 -> Moments of inertia/16(r6)
  Demux1/4 -> Moments of inertia/10(r4)
  Demux1/1 -> Moments of inertia/1(r1)
  Demux/1 -> Moments of inertia/3(m1)
  M(q),C(q,dq),g(q)/4(M) -> F gen./1(M)
  Moments of inertia/3(I3) -> M(q),C(q,dq),g(q)/5(I3)
  M(q),C(q,dq),g(q)/5(H) -> F gen./2(H)
  Clock/1 -> To Workspace35/1
  Z/12(w6) -> To Workspace31/1, M(q),C(q,dq),g(q)/14(w6)
  Demux2/2 -> Moments of inertia/5(h2)
  H_6^0/7(R_6^0) -> To Workspace18/1, Jacobian/6(R_6^0)
  H_6^0/1(H_6^0) -> To Workspace/1, Display1/1
  Demux1/3 -> Moments of inertia/7(r3)
  Z/6(v6) -> To Workspace12/1
  Moments of inertia/6(I6) -> M(q),C(q,dq),g(q)/8(I6)
  Z/4(v4) -> To Workspace10/1
  Demux2/5 -> Moments of inertia/14(h5)
  H_6^0/9(p_2^0) -> To Workspace23/1, Jacobian/8(p_2^0)
  H_6^0/13(p_6^0) -> To Workspace22/1, Jacobian/12(p_6^0)
  Demux2/4 -> Moments of inertia/11(h4)
  Demux/3 -> Moments of inertia/9(m3)
  H_6^0/10(p_3^0) -> Jacobian/9(p_3^0), To Workspace19/1
  Z/7(w1) -> To Workspace25/1, M(q),C(q,dq),g(q)/9(w1)
  Demux2/3 -> Moments of inertia/8(h3)
  H_6^0/6(R_5^0) -> To Workspace17/1, Jacobian/5(R_5^0)
  Sum/1 -> To Workspace34/1, Dynamics/5(tau)
  dq(0)/1 -> Dynamics/7(dq0)
  q(0)/1 -> Dynamics/6(q0)
  M(q),C(q,dq),g(q)/2(C(q,dq)) -> Slotine/2(C(q,dq)), To Workspace4/1, Dynamics/2(C(q,dq))
  H_6^0/11(p_4^0) -> To Workspace20/1, Jacobian/10(p_4^0)
  M(q),C(q,dq),g(q)/6(G) -> F gen./3(G)
  Z/2(v2) -> To Workspace7/1
  Z/9(w3) -> To Workspace28/1, M(q),C(q,dq),g(q)/11(w3)
  H_6^0/8(p_1^0) -> Jacobian/7(p_1^0), To Workspace24/1
  Demux2/1 -> Moments of inertia/2(h1)
  H_6^0/5(R_4^0) -> To Workspace16/1, Jacobian/4(R_4^0)
  Type: Revolute/1 -> Jacobian/14(type2), Jacobian/15(type3), Jacobian/18(type6), Jacobian/17(type5), Jacobian/16(type4), Jacobian/13(type1)
  Z/1(v1) -> To Workspace6/1
  Z/5(v5) -> To Workspace11/1
  tau(t)/1(tau) -> Gain/1
  Jacobian/2(J(q)) -> Z/1(J(q)), M(q),C(q,dq),g(q)/2(J(q)), To Workspace2/1
  H_6^0/12(p_5^0) -> To Workspace21/1, Jacobian/11(p_5^0)
  F gen./1(F) -> To Workspace33/1
  Dynamics/1(q+delta_q) -> q+delta_q/1, Scope1/1, To Workspace9/1, Slotine/7(q), H_6^0/3(theta)
  Demux/2 -> Moments of inertia/6(m2)
  Moments of inertia/1(I1) -> M(q),C(q,dq),g(q)/3(I1)
  a/1 -> H_6^0/1(a)
  d/1 -> H_6^0/4(d)
  Moments of inertia/2(I2) -> M(q),C(q,dq),g(q)/4(I2)
  Dynamics/2(dq+delta_dq) -> Scope/1, To Workspace32/1, Z/2(dq), Slotine/8(dq), Dynamics/4(dq)
  Z/10(w4) -> To Workspace29/1, M(q),C(q,dq),g(q)/12(w4)
  Z/8(w2) -> To Workspace27/1, M(q),C(q,dq),g(q)/10(w2)
  Constant1/1 -> Slotine/10(K)
  Demux1/2 -> Moments of inertia/4(r2)
  Demux1/5 -> Moments of inertia/13(r5)
  Moments of inertia/4(I4) -> M(q),C(q,dq),g(q)/6(I4)
  H_6^0/4(R_3^0) -> To Workspace15/1, Jacobian/3(R_3^0)
  Derivative/1 -> To Workspace26/1
  Z/11(w5) -> To Workspace30/1, M(q),C(q,dq),g(q)/13(w5)
  alpha/1 -> H_6^0/2(alpha)
  H_6^0/2(R_1^0) -> To Workspace13/1, Jacobian/1(R_1^0)
  q_d/1 -> Slotine/4(q_d)
  Demux/6 -> Moments of inertia/18(m6)
  M(q),C(q,dq),g(q)/3(M(q)) -> Slotine/3(M(q)), To Workspace5/1, Derivative/1, Dynamics/1(M(q))

== system ROBOT_OK/Subsystem2/Dynamics ==
  M(q) : Inport
  C(q,dq) : Inport  Port=2
  g(q) : Inport  Port=3
  dq : Inport  Port=4
  tau : Inport  Port=5
  q0 : Inport  Port=6
  dq0 : Inport  Port=7
  Add : Sum
  Add1 : Sum
  Band-Limited White Noise : simulink/Sources/Band-Limited White Noise  Cov=[0.1]  Ts=0.001  seed=[23341]
  Friction : Subsystem
  Gain : Gain  Gain=-1
  Gain1 : Gain
  Gain2 : Gain
  "Integrator, Second-Order" : SecondOrderIntegrator  ICSourceX=external  ICSourceDXDT=external
  Interpreted MATLAB Function : MATLABFcn  MATLABFcn=inv  OutputSignalType=real  Output1D=off
  Product : Product  Multiplication=Matrix(*)
  Product1 : Product  Multiplication=Matrix(*)
  Saturation : Saturate  UpperLimit=30  LowerLimit=-30
  Saturation1 : Saturate  UpperLimit=1  LowerLimit=-1
  Sum : Sum  Inputs=|++
  q+delta_q : Outport
  dq+delta_dq : Outport  Port=2
  ddq+delta_ddq : Outport  Port=3
  tau_f_2 : Outport  Port=4
  wires:
  C(q,dq)/1 -> Product/1
  dq/1 -> Product/2
  Product/1 -> Add/1
  g(q)/1 -> Add/2
  Add/1 -> Gain/1
  M(q)/1 -> Interpreted MATLAB Function/1
  Interpreted MATLAB Function/1 -> Product1/1
  Gain/1 -> Add1/1
  tau/1 -> Saturation/1
  Add1/1 -> Product1/2
  Product1/1 -> ddq+delta_ddq/1, "Integrator, Second-Order"/1
  "Integrator, Second-Order"/2 -> Friction/1(dq), dq+delta_dq/1
  "Integrator, Second-Order"/1 -> q+delta_q/1
  q0/1 -> "Integrator, Second-Order"/2
  dq0/1 -> "Integrator, Second-Order"/3
  Sum/1 -> Add1/2
  Saturation/1 -> Sum/1
  Friction/1(tau_f) -> Gain1/1, tau_f_2/1
  Band-Limited White Noise/1 -> Gain2/1
  Saturation1/1 -> Friction/2(d(t))
  Gain1/1 -> Sum/2
  Gain2/1 -> Saturation1/1

== system ROBOT_OK/Subsystem2/F gen. ==
  M : Inport
  H : Inport  Port=2
  G : Inport  Port=3
  Z : Inport  Port=4
  Add : Sum  Inputs=+++
  Derivative : Derivative
  Product1 : Product  Multiplication=Matrix(*)
  Product2 : Product  Multiplication=Matrix(*)
  F : Outport
  wires:
  Z/1 -> Product1/2, Derivative/1
  Add/1 -> F/1
  G/1 -> Add/3
  Product2/1 -> Add/1
  M/1 -> Product2/1
  Derivative/1 -> Product2/2
  Product1/1 -> Add/2
  H/1 -> Product1/1

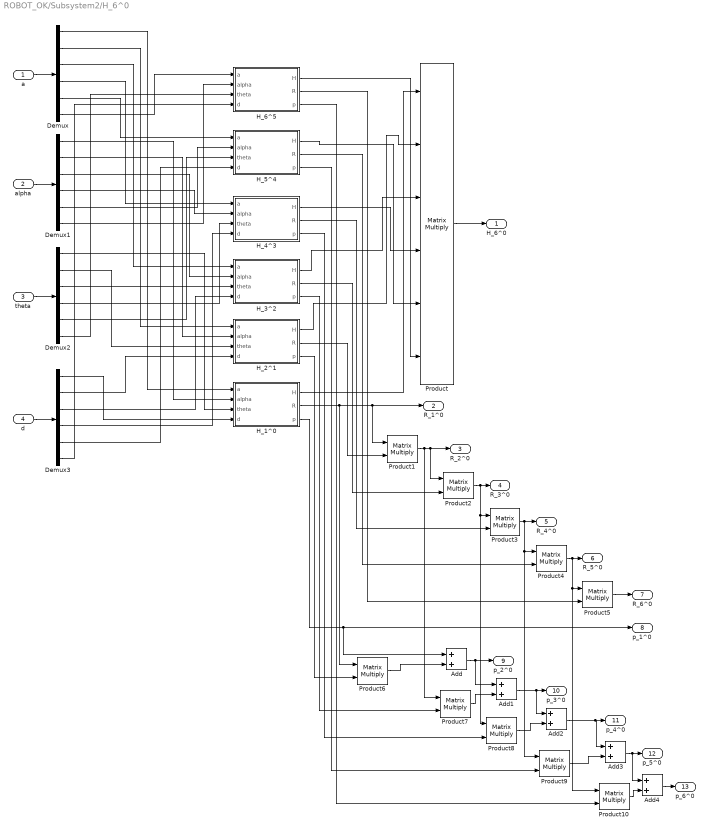
== system ROBOT_OK/Subsystem2/H_6^0 ==
  a : Inport
  alpha : Inport  Port=2
  theta : Inport  Port=3
  d : Inport  Port=4
  Add{,1..4} (5 alike) : Sum
  Demux{,1..3} (4 alike) : Demux  Outputs=6
  H_1^0 : Subsystem
  H_2^1 : Subsystem
  H_3^2 : Subsystem
  H_4^3 : Subsystem
  H_5^4 : Subsystem
  H_6^5 : Subsystem
  Product : Product  Inputs=6  Multiplication=Matrix(*)
  Product{1..10} (10 alike) : Product  Multiplication=Matrix(*)
  H_6^0 : Outport
  R_1^0 : Outport  Port=2
  R_2^0 : Outport  Port=3
  R_3^0 : Outport  Port=4
  R_4^0 : Outport  Port=5
  R_5^0 : Outport  Port=6
  R_6^0 : Outport  Port=7
  p_1^0 : Outport  Port=8
  p_2^0 : Outport  Port=9
  p_3^0 : Outport  Port=10
  p_4^0 : Outport  Port=11
  p_5^0 : Outport  Port=12
  p_6^0 : Outport  Port=13
  wires:
  H_6^5/1(H) -> Product/6
  H_5^4/1(H) -> Product/5
  H_2^1/1(H) -> Product/2
  H_1^0/1(H) -> Product/1
  Product/1 -> H_6^0/1
  a/1 -> Demux/1
  d/1 -> Demux3/1
  H_4^3/1(H) -> Product/4
  H_3^2/1(H) -> Product/3
  Product1/1 -> Product7/1, Product2/1, R_2^0/1
  H_2^1/2(R) -> Product1/2
  Product2/1 -> Product8/1, Product3/1, R_3^0/1
  Product3/1 -> Product9/1, Product4/1, R_4^0/1
  Product4/1 -> Product10/1, Product5/1, R_5^0/1
  Product5/1 -> R_6^0/1
  Add/1 -> Add1/1, p_2^0/1
  theta/1 -> Demux2/1
  alpha/1 -> Demux1/1
  Demux/1 -> H_1^0/1(a)
  Demux/6 -> H_6^5/1(a)
  Demux/5 -> H_5^4/1(a)
  Demux/4 -> H_4^3/1(a)
  Demux/3 -> H_3^2/1(a)
  Demux/2 -> H_2^1/1(a)
  Demux1/6 -> H_6^5/2(alpha)
  Demux1/5 -> H_5^4/2(alpha)
  Demux1/4 -> H_4^3/2(alpha)
  Demux1/3 -> H_3^2/2(alpha)
  Demux1/2 -> H_2^1/2(alpha)
  Demux1/1 -> H_1^0/2(alpha)
  Demux2/6 -> H_6^5/3(theta)
  Demux2/5 -> H_5^4/3(theta)
  Demux2/4 -> H_4^3/3(theta)
  Demux2/3 -> H_3^2/3(theta)
  Demux2/2 -> H_2^1/3(theta)
  Demux2/1 -> H_1^0/3(theta)
  Demux3/1 -> H_1^0/4(d)
  Demux3/2 -> H_2^1/4(d)
  Demux3/3 -> H_3^2/4(d)
  Demux3/4 -> H_4^3/4(d)
  Demux3/5 -> H_5^4/4(d)
  Demux3/6 -> H_6^5/4(d)
  H_3^2/2(R) -> Product2/2
  H_4^3/2(R) -> Product3/2
  H_5^4/2(R) -> Product4/2
  H_6^5/2(R) -> Product5/2
  H_1^0/3(p) -> Add/1, p_1^0/1
  H_2^1/3(p) -> Product6/2
  Add1/1 -> Add2/1, p_3^0/1
  H_3^2/3(p) -> Product7/2
  H_4^3/3(p) -> Product8/2
  Add2/1 -> Add3/1, p_4^0/1
  H_5^4/3(p) -> Product9/2
  Add3/1 -> Add4/1, p_5^0/1
  H_6^5/3(p) -> Product10/2
  Add4/1 -> p_6^0/1
  H_1^0/2(R) -> R_1^0/1, Product1/1, Product6/1
  Product6/1 -> Add/2
  Product7/1 -> Add1/2
  Product8/1 -> Add2/2
  Product9/1 -> Add3/2
  Product10/1 -> Add4/2

== system ROBOT_OK/Subsystem2/Jacobian ==
  R_1^0 : Inport
  R_2^0 : Inport  Port=2
  R_3^0 : Inport  Port=3
  R_4^0 : Inport  Port=4
  R_5^0 : Inport  Port=5
  R_6^0 : Inport  Port=6
  p_1^0 : Inport  Port=7
  p_2^0 : Inport  Port=8
  p_3^0 : Inport  Port=9
  p_4^0 : Inport  Port=10
  p_5^0 : Inport  Port=11
  p_6^0 : Inport  Port=12
  type1 : Inport  Port=13
  type2 : Inport  Port=14
  type3 : Inport  Port=15
  type4 : Inport  Port=16
  type5 : Inport  Port=17
  type6 : Inport  Port=18
  J(q) gen. : Subsystem
  J_v : Subsystem
  J_w : Subsystem
  Vector Concatenate : Concatenate  Mode=Multidimensional array
  J : Outport
  J(q) : Outport  Port=2
  wires:
  R_1^0/1 -> J_v/1(R_1^0), J_w/1(R_1^0), J(q) gen./1(R_1^0)
  p_1^0/1 -> J_v/7(p_1^0), J(q) gen./7(p_1^0)
  p_2^0/1 -> J_v/8(p_2^0), J(q) gen./8(p_2^0)
  p_3^0/1 -> J_v/9(p_3^0), J(q) gen./9(p_3^0)
  p_4^0/1 -> J_v/10(p_4^0), J(q) gen./10(p_4^0)
  p_5^0/1 -> J_v/11(p_5^0), J(q) gen./11(p_5^0)
  R_2^0/1 -> J_v/2(R_2^0), J_w/2(R_2^0), J(q) gen./2(R_2^0)
  R_3^0/1 -> J_v/3(R_3^0), J_w/3(R_3^0), J(q) gen./3(R_3^0)
  R_4^0/1 -> J_v/4(R_4^0), J_w/4(R_4^0), J(q) gen./4(R_4^0)
  R_5^0/1 -> J_v/5(R_5^0), J_w/5(R_5^0), J(q) gen./5(R_5^0)
  type1/1 -> J_w/7(type1), J_v/13(type1), J(q) gen./12(type1)
  type2/1 -> J_w/8(type2), J(q) gen./13(type2), J_v/14(type2)
  type3/1 -> J_w/9(type3), J(q) gen./14(type3), J_v/15(type3)
  type4/1 -> J_w/10(type4), J(q) gen./15(type4), J_v/16(type4)
  type5/1 -> J_w/11(type5), J_v/17(type5)
  type6/1 -> J_w/12(type6), J_v/18(type6)
  p_6^0/1 -> J_v/12(p_6^0)
  J_v/1(J_v) -> J(q) gen./16(J_v_6(q)), Vector Concatenate/1
  J_w/1(EF J_w) -> Vector Concatenate/2
  Vector Concatenate/1 -> J/1
  J(q) gen./1(J(q)) -> J(q)/1
  J_w/2(J_w1) -> J(q) gen./17(J_w1)
  J_w/3(J_w2) -> J(q) gen./18(J_w2)
  J_w/4(J_w3) -> J(q) gen./19(J_w3)
  J_w/5(J_w4) -> J(q) gen./20(J_w4)
  J_w/6(J_w5) -> J(q) gen./21(J_w5)
  J_w/7(J_w6) -> J(q) gen./22(J_w6)
  R_6^0/1 -> J_v/6(R_6^0), J_w/6(R_6^0), J(q) gen./6(R_6^0)

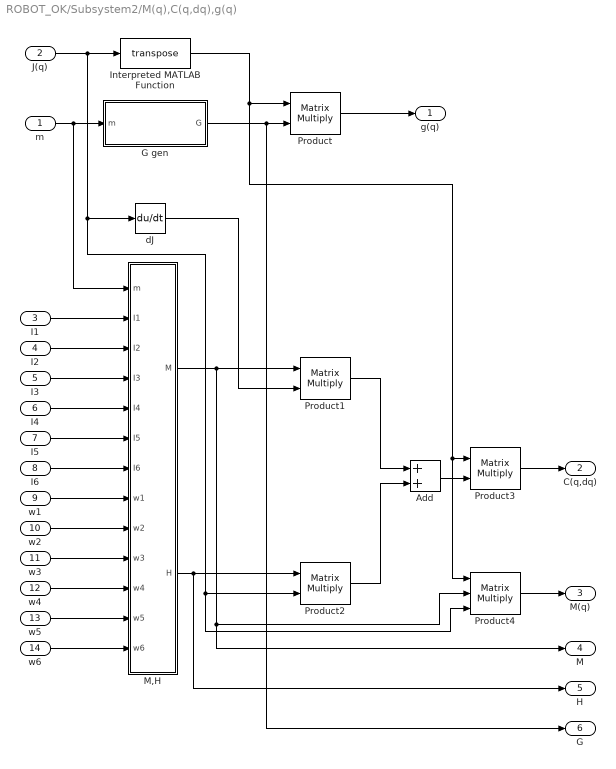
== system ROBOT_OK/Subsystem2/M(q),C(q,dq),g(q) ==
  m : Inport
  J(q) : Inport  Port=2
  I1 : Inport  Port=3
  I2 : Inport  Port=4
  I3 : Inport  Port=5
  I4 : Inport  Port=6
  I5 : Inport  Port=7
  I6 : Inport  Port=8
  w1 : Inport  Port=9
  w2 : Inport  Port=10
  w3 : Inport  Port=11
  w4 : Inport  Port=12
  w5 : Inport  Port=13
  w6 : Inport  Port=14
  Add : Sum
  G gen : Subsystem
  Interpreted MATLAB Function : MATLABFcn  MATLABFcn=transpose  OutputSignalType=real  Output1D=off
  M,H : Subsystem
  Product{,1..3} (4 alike) : Product  Multiplication=Matrix(*)
  Product4 : Product  Inputs=3  Multiplication=Matrix(*)
  dJ : Derivative
  g(q) : Outport
  C(q,dq) : Outport  Port=2
  M(q) : Outport  Port=3
  M : Outport  Port=4
  H : Outport  Port=5
  G : Outport  Port=6
  wires:
  J(q)/1 -> Interpreted MATLAB Function/1, Product4/3, Product2/2, dJ/1
  Interpreted MATLAB Function/1 -> Product4/1, Product3/1, Product/1
  Product/1 -> g(q)/1
  m/1 -> G gen/1(m), M,H/1(m)
  I1/1 -> M,H/2(I1)
  I2/1 -> M,H/3(I2)
  I3/1 -> M,H/4(I3)
  I4/1 -> M,H/5(I4)
  I5/1 -> M,H/6(I5)
  I6/1 -> M,H/7(I6)
  w1/1 -> M,H/8(w1)
  w2/1 -> M,H/9(w2)
  w3/1 -> M,H/10(w3)
  w4/1 -> M,H/11(w4)
  w5/1 -> M,H/12(w5)
  w6/1 -> M,H/13(w6)
  M,H/1(M) -> Product1/1, M/1, Product4/2
  dJ/1 -> Product1/2
  M,H/2(H) -> H/1, Product2/1
  Product1/1 -> Add/1
  Product2/1 -> Add/2
  Add/1 -> Product3/2
  Product3/1 -> C(q,dq)/1
  Product4/1 -> M(q)/1
  G gen/1(G) -> G/1, Product/2

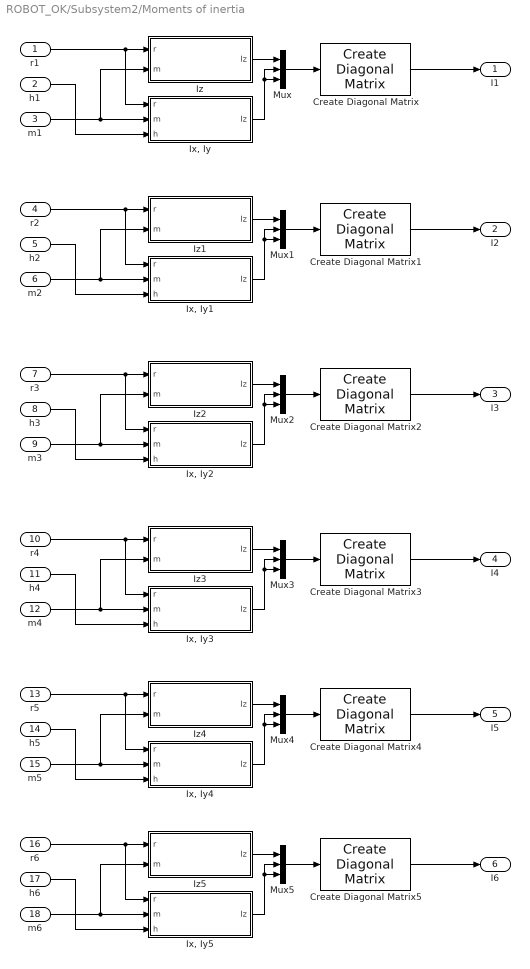
== system ROBOT_OK/Subsystem2/Moments of inertia ==
  r1 : Inport
  h1 : Inport  Port=2
  m1 : Inport  Port=3
  r2 : Inport  Port=4
  h2 : Inport  Port=5
  m2 : Inport  Port=6
  r3 : Inport  Port=7
  h3 : Inport  Port=8
  m3 : Inport  Port=9
  r4 : Inport  Port=10
  h4 : Inport  Port=11
  m4 : Inport  Port=12
  r5 : Inport  Port=13
  h5 : Inport  Port=14
  m5 : Inport  Port=15
  r6 : Inport  Port=16
  h6 : Inport  Port=17
  m6 : Inport  Port=18
  Create Diagonal Matrix{,1..5} (6 alike) : dspmtrx3/Create Diagonal Matrix
      settings: SourceProductBaseCode=DS
  "Ix, Iy" : Subsystem
  "Ix, Iy1" : Subsystem
  "Ix, Iy2" : Subsystem
  "Ix, Iy3" : Subsystem
  "Ix, Iy4" : Subsystem
  "Ix, Iy5" : Subsystem
  Iz : Subsystem
  Iz1 : Subsystem
  Iz2 : Subsystem
  Iz3 : Subsystem
  Iz4 : Subsystem
  Iz5 : Subsystem
  Mux{,1..5} (6 alike) : Mux  Inputs=3
  I1 : Outport
  I2 : Outport  Port=2
  I3 : Outport  Port=3
  I4 : Outport  Port=4
  I5 : Outport  Port=5
  I6 : Outport  Port=6
  wires:
  r1/1 -> "Ix, Iy"/1(r), Iz/1(r)
  m1/1 -> "Ix, Iy"/2(m), Iz/2(m)
  h1/1 -> "Ix, Iy"/3(h)
  Mux/1 -> Create Diagonal Matrix/1
  Iz/1(Iz) -> Mux/1
  "Ix, Iy"/1(Iz) -> Mux/3, Mux/2
  Create Diagonal Matrix/1 -> I1/1
  r2/1 -> "Ix, Iy1"/1(r), Iz1/1(r)
  m2/1 -> "Ix, Iy1"/2(m), Iz1/2(m)
  h2/1 -> "Ix, Iy1"/3(h)
  Mux1/1 -> Create Diagonal Matrix1/1
  Iz1/1(Iz) -> Mux1/1
  "Ix, Iy1"/1(Iz) -> Mux1/3, Mux1/2
  Create Diagonal Matrix1/1 -> I2/1
  r3/1 -> "Ix, Iy2"/1(r), Iz2/1(r)
  m3/1 -> "Ix, Iy2"/2(m), Iz2/2(m)
  h3/1 -> "Ix, Iy2"/3(h)
  Mux2/1 -> Create Diagonal Matrix2/1
  Iz2/1(Iz) -> Mux2/1
  "Ix, Iy2"/1(Iz) -> Mux2/3, Mux2/2
  Create Diagonal Matrix2/1 -> I3/1
  r4/1 -> "Ix, Iy3"/1(r), Iz3/1(r)
  m4/1 -> "Ix, Iy3"/2(m), Iz3/2(m)
  h4/1 -> "Ix, Iy3"/3(h)
  Mux3/1 -> Create Diagonal Matrix3/1
  Iz3/1(Iz) -> Mux3/1
  "Ix, Iy3"/1(Iz) -> Mux3/3, Mux3/2
  Create Diagonal Matrix3/1 -> I4/1
  r5/1 -> "Ix, Iy4"/1(r), Iz4/1(r)
  m5/1 -> "Ix, Iy4"/2(m), Iz4/2(m)
  h5/1 -> "Ix, Iy4"/3(h)
  Mux4/1 -> Create Diagonal Matrix4/1
  Iz4/1(Iz) -> Mux4/1
  "Ix, Iy4"/1(Iz) -> Mux4/3, Mux4/2
  Create Diagonal Matrix4/1 -> I5/1
  r6/1 -> "Ix, Iy5"/1(r), Iz5/1(r)
  m6/1 -> "Ix, Iy5"/2(m), Iz5/2(m)
  h6/1 -> "Ix, Iy5"/3(h)
  Mux5/1 -> Create Diagonal Matrix5/1
  Iz5/1(Iz) -> Mux5/1
  "Ix, Iy5"/1(Iz) -> Mux5/3, Mux5/2
  Create Diagonal Matrix5/1 -> I6/1

== system ROBOT_OK/Subsystem2/Slotine ==
  g(q) : Inport
  C(q,dq) : Inport  Port=2
  M(q) : Inport  Port=3
  q_d : Inport  Port=4
  dq_d : Inport  Port=5
  ddq_d : Inport  Port=6
  q : Inport  Port=7
  dq : Inport  Port=8
  Lambda : Inport  Port=9
  K : Inport  Port=10
  Clock : Clock
  Gain : Gain  Gain=-1
  Math Function : Math  SignedPower=on  SaturateOnIntegerOverflow=on
  S-gen : Subsystem
  V-gen : Subsystem
  dV-gen : Subsystem
  dq_tilde : Sum  Inputs=-+
  q_tilde : Sum  Inputs=-+
  tau-gen : Subsystem
  u0-gen : Subsystem
  tau : Outport
  S : Outport  Port=2
  wires:
  q_d/1 -> q_tilde/1
  q/1 -> q_tilde/2
  dq_d/1 -> V-gen/2(dq_d), dq_tilde/1
  dq/1 -> S-gen/1(dq), dq_tilde/2
  ddq_d/1 -> dV-gen/2(ddq_d)
  q_tilde/1 -> V-gen/1(q_tilde)
  Lambda/1 -> dV-gen/3(Gamma), V-gen/3(Gamma)
  dq_tilde/1 -> dV-gen/1(dq_tilde)
  V-gen/1(V) -> tau-gen/4(V), S-gen/2(V)
  M(q)/1 -> tau-gen/1(M)
  C(q,dq)/1 -> tau-gen/2(C)
  g(q)/1 -> tau-gen/3(g)
  dV-gen/1(dV) -> tau-gen/5(dV)
  S-gen/1(S) -> u0-gen/1(S), S/1, tau-gen/6(S)
  K/1 -> tau-gen/7(K)
  tau-gen/1(tau) -> tau/1
  u0-gen/1(u0) -> tau-gen/8(u0)
  Math Function/1 -> u0-gen/2(sigma(t))
  Clock/1 -> Gain/1
  Gain/1 -> Math Function/1

== system ROBOT_OK/Subsystem2/Z ==
  J(q) : Inport
  dq : Inport  Port=2
  Demux : Demux  Outputs=36
  Mux{,1..11} (12 alike) : Mux  Inputs=3
  Product : Product  Multiplication=Matrix(*)
  v1 : Outport
  v2 : Outport  Port=2
  v3 : Outport  Port=3
  v4 : Outport  Port=4
  v5 : Outport  Port=5
  v6 : Outport  Port=6
  w1 : Outport  Port=7
  w2 : Outport  Port=8
  w3 : Outport  Port=9
  w4 : Outport  Port=10
  w5 : Outport  Port=11
  w6 : Outport  Port=12
  Z : Outport  Port=13
  wires:
  J(q)/1 -> Product/1
  dq/1 -> Product/2
  Product/1 -> Z/1, Demux/1
  Demux/1 -> Mux/1
  Demux/2 -> Mux/2
  Demux/3 -> Mux/3
  Mux/1 -> v1/1
  Demux/4 -> Mux1/1
  Demux/5 -> Mux1/2
  Demux/6 -> Mux1/3
  Mux1/1 -> v2/1
  Mux2/1 -> v3/1
  Demux/7 -> Mux2/1
  Demux/8 -> Mux2/2
  Demux/9 -> Mux2/3
  Mux3/1 -> v4/1
  Demux/10 -> Mux3/1
  Demux/11 -> Mux3/2
  Demux/12 -> Mux3/3
  Mux4/1 -> v5/1
  Demux/14 -> Mux4/2
  Demux/13 -> Mux4/1
  Demux/15 -> Mux4/3
  Mux5/1 -> v6/1
  Demux/17 -> Mux5/2
  Demux/16 -> Mux5/1
  Demux/18 -> Mux5/3
  Mux6/1 -> w1/1
  Demux/19 -> Mux6/1
  Demux/20 -> Mux6/2
  Demux/21 -> Mux6/3
  Mux7/1 -> w2/1
  Demux/22 -> Mux7/1
  Demux/23 -> Mux7/2
  Demux/24 -> Mux7/3
  Mux8/1 -> w3/1
  Demux/25 -> Mux8/1
  Demux/26 -> Mux8/2
  Demux/27 -> Mux8/3
  Mux9/1 -> w4/1
  Demux/28 -> Mux9/1
  Demux/29 -> Mux9/2
  Demux/30 -> Mux9/3
  Mux10/1 -> w5/1
  Demux/31 -> Mux10/1
  Demux/32 -> Mux10/2
  Demux/33 -> Mux10/3
  Mux11/1 -> w6/1
  Demux/34 -> Mux11/1
  Demux/35 -> Mux11/2
  Demux/36 -> Mux11/3

== system ROBOT_OK/Subsystem2/tau(t) ==
  g(q) : Inport
  Add : Sum
  Constant : Constant  Value=zeros(5,1)
  Gain : Gain  Gain=0
  Mux : Mux  Inputs=2
  Sine Wave : Sin  SampleTime=0
  tau : Outport
  wires:
  Sine Wave/1 -> Mux/2
  Constant/1 -> Mux/1
  Add/1 -> tau/1
  Mux/1 -> Gain/1
  g(q)/1 -> Add/1
  Gain/1 -> Add/2

== system ROBOT_OK/Subsystem3/ROBOT_ARM_1004_1_RIGID ==
  ReferenceFrame : sm_lib/Frames and Transforms/Reference Frame
  Solid : sm_lib/Body Elements/File Solid  ExtGeomFileName=ROBOT_ARM_1004_Predeterminado_sldprt.STEP  UnitType=FromFile  ExtGeomFileUnits=m  StepReaderType=HEX  ExportConvexHullGeometry=off  InertiaType=Custom  Mass=smiData.Solid(5).mass  MassUnits=kg  CenterOfMass=smiData.Solid(5).CoM  CenterOfMassUnits=mm  MomentsOfInertia=smiData.Solid(5).MoI  MomentsOfInertiaUnits=kg*mm^2  ProductsOfInertia=smiData.Solid(5).PoI  ProductsOfInertiaUnits=kg*mm^2  BasedOnType=DensityFromFile  Density=1000  DensityUnits=kg/m^3  DoExposeReferenceFrame=on  SerializedFrames=<Frames/>  GraphicType=FromGeometry  MarkerShape=Sphere  MarkerSize=10  GraphicVisPropType=SimpleVisualProperties  GraphicDiffuseColor=smiData.Solid(5).color  GraphicSpecularColor=[0.5 0.5 0.5 1.0]  GraphicAmbientColor=[0.15 0.15 0.15 1.0]  GraphicEmissiveColor=[0.0 0.0 0.0 1.0]  GraphicShininess=75  GraphicOpacity=smiData.Solid(5).opacity
  Transform : sm_lib/Frames and Transforms/Rigid Transform  TranslationMethod=Cartesian  TranslationStandardOffset=0  TranslationLengthUnit=mm  TranslationStandardAxis=+Z  TranslationCartesianOffset=smiData.RigidTransform(8).translation  TranslationROffset=0  TranslationROffsetUnits=m  TranslationZOffset=0  TranslationZOffsetUnits=m  TranslationThetaOffset=0  TranslationThetaOffsetUnits=deg  RotationMethod=ArbitraryAxis  RotationAngleUnits=rad  RotationStandardAxis=+Z  RotationAngle=smiData.RigidTransform(8).angle  RotationArbitraryAxis=smiData.RigidTransform(8).axis  FollAlignAxisA=+X  BaseAlignAxisA=+Y  FollAlignAxisB=+Y  BaseAlignAxisB=+Z  RotationSequenceAxes=FollowerAxes  RotationSequence=XYX  RotationSequenceAngles=[0 0 0]  RotationSequenceAnglesUnits=deg  RotationMatrix=[1 0 0; 0 1 0; 0 0 1]
  Transform1 : sm_lib/Frames and Transforms/Rigid Transform  TranslationMethod=Cartesian  TranslationStandardOffset=0  TranslationLengthUnit=mm  TranslationStandardAxis=+Z  TranslationCartesianOffset=smiData.RigidTransform(11).translation  TranslationROffset=0  TranslationROffsetUnits=m  TranslationZOffset=0  TranslationZOffsetUnits=m  TranslationThetaOffset=0  TranslationThetaOffsetUnits=deg  RotationMethod=ArbitraryAxis  RotationAngleUnits=rad  RotationStandardAxis=+Z  RotationAngle=smiData.RigidTransform(11).angle  RotationArbitraryAxis=smiData.RigidTransform(11).axis  FollAlignAxisA=+X  BaseAlignAxisA=+Y  FollAlignAxisB=+Y  BaseAlignAxisB=+Z  RotationSequenceAxes=FollowerAxes  RotationSequence=XYX  RotationSequenceAngles=[0 0 0]  RotationSequenceAnglesUnits=deg  RotationMatrix=[1 0 0; 0 1 0; 0 0 1]
  F : PMIOPort  Side=Left
  F1 : PMIOPort  Port=2  Side=Right
  connections:
  ReferenceFrame/RConn1 -- Solid/RConn1 -- Transform/LConn1 -- Transform1/LConn1
  Transform/RConn1 -- F/RConn1
  Transform1/RConn1 -- F1/RConn1
